simulink model "Bioinspired_backstepping_control"  (R2021b)
settings: Solver=FixedStepAuto  StartTime=0.0  StopTime=10  FixedStep=0.01  RelTol=1e-3
settings Model: Creator=chane  LastModifiedBy=jayeshjayashankar

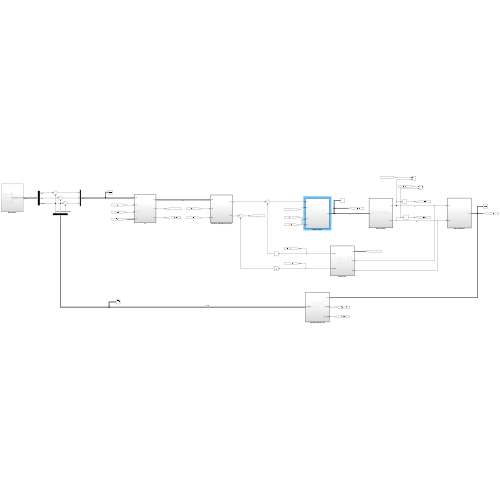
[thumbnail: Simulink's stored preview of the top-level diagram]
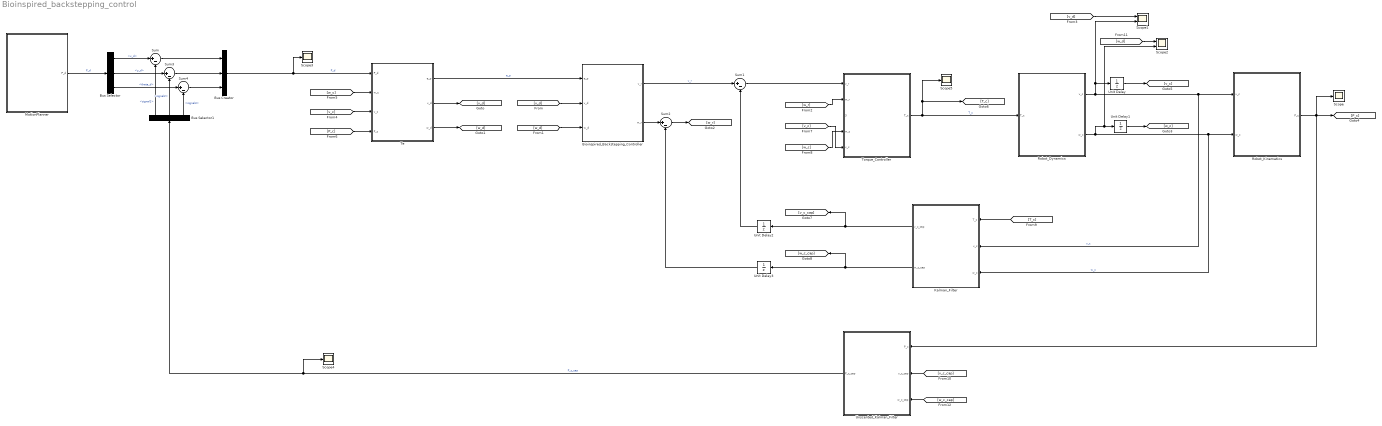
== system Bioinspired_backstepping_control ==
  Bioinspired_Backstepping_Controller : Subsystem  TreatAsAtomicUnit=on
  Bus Creator : BusCreator  Inputs=3
  Bus Selector : BusSelector  OutputSignals=x_d,y_d,theta_d
  Bus Selector1 : BusSelector  OutputSignals=signal1,signal2,signal3
  Kalman_Filter : Subsystem  TreatAsAtomicUnit=on
  MotionPlanner : Subsystem
  Robot_Dynamics : Subsystem  TreatAsAtomicUnit=on
      settings: MinAlgLoopOccurrences=on
  Robot_Kinematics : Subsystem  TreatAsAtomicUnit=on
      settings: MinAlgLoopOccurrences=on
  Scope{,3..5} (4 alike) : Scope
  Scope1 : Scope  NumInputPorts=2
  Scope2 : Scope  NumInputPorts=2
  Sum{,1..4} (5 alike) : Sum  Inputs=|+-
  Te : Subsystem  TreatAsAtomicUnit=on
  Torque_Controller : Subsystem  TreatAsAtomicUnit=on
  Unit Delay{,1..3} (4 alike) : UnitDelay  SampleTime=-1  HasFrameUpgradeWarning=on
  Unscented_Kalman_Filter : Subsystem  TreatAsAtomicUnit=on
      settings: MinAlgLoopOccurrences=on
  wires:
  Te/1(e_p) -> Bioinspired_Backstepping_Controller/1(e_p)  "e_p"
  Te/2(v_d) -> [v_d]
  [v_d] -> Bioinspired_Backstepping_Controller/2(v_d)
  Te/3(w_d) -> [w_d]
  [w_d] -> Bioinspired_Backstepping_Controller/3(w_d)
  [w_r] -> Torque_Controller/2(w_r)
  Torque_Controller/1(T_c) -> Scope5/1, [T_c], Robot_Dynamics/1(T_c)  "T_c"
  Robot_Dynamics/1(v_c) -> Kalman_Filter/2(v_c), Robot_Kinematics/1(v_c), Scope1/2, Unit Delay/1  "v_c"
  [v_c] -> Te/3(v_c)
  [w_c] -> Te/2(w_c)
  [P_c] -> Te/4(P_c)
  [v_c] -> Torque_Controller/5(v_c)
  [w_c] -> Torque_Controller/4(w_c)
  [T_c] -> Kalman_Filter/1(T_c)
  Robot_Dynamics/2(w_c) -> Kalman_Filter/3(w_c), Robot_Kinematics/2(w_c), Scope2/2, Unit Delay1/1  "w_c"
  Bioinspired_Backstepping_Controller/1(v_r) -> Sum1/1  "v_r"
  Sum1/1 -> Torque_Controller/1(v_r)
  Kalman_Filter/1(v_c_cap) -> [v_c_cap], Unit Delay2/1
  Kalman_Filter/2(w_c_cap) -> [w_c_cap], Unit Delay3/1
  [v_c_cap] -> Unscented_Kalman_Filter/2(v_c_cap)
  [w_c_cap] -> Unscented_Kalman_Filter/3(w_c_cap)
  Unscented_Kalman_Filter/1(P_c_cap) -> Scope4/1, Bus Selector1/1  "P_c_cap"
  MotionPlanner/1(P_d) -> Bus Selector/1  "P_d"
  Bus Selector/1 -> Sum/1  "<x_d>"
  Bus Selector1/1 -> Sum/2  "<signal1>"
  Sum/1 -> Bus Creator/1
  Bus Selector/2 -> Sum3/1  "<y_d>"
  Bus Selector1/2 -> Sum3/2  "<signal2>"
  Sum3/1 -> Bus Creator/2
  Bus Selector1/3 -> Sum4/2  "<signal3>"
  Bus Selector/3 -> Sum4/1  "<theta_d>"
  Sum4/1 -> Bus Creator/3
  Bus Creator/1 -> Scope3/1, Te/1(P_d)  "P_d"
  Unit Delay/1 -> [v_c]
  Unit Delay1/1 -> [w_c]
  Robot_Kinematics/1(P_c) -> Unscented_Kalman_Filter/1(P_c), Scope/1, [P_c]
  Unit Delay2/1 -> Sum1/2
  Unit Delay3/1 -> Sum2/2
  [v_d] -> Scope1/1
  [w_d] -> Scope2/1
  Bioinspired_Backstepping_Controller/2(w_r) -> Sum2/1
  Sum2/1 -> [w_r]

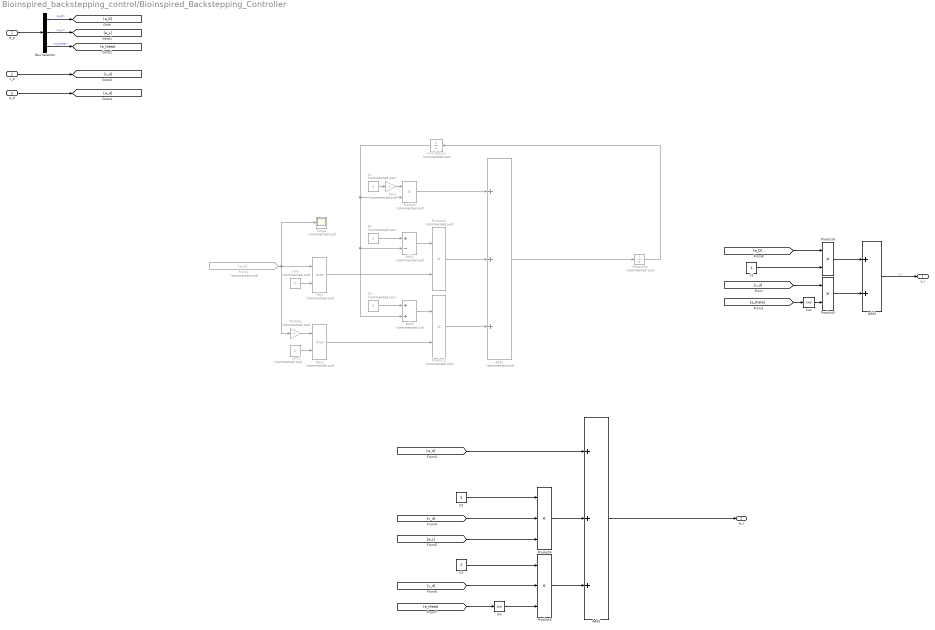
== system Bioinspired_backstepping_control/Bioinspired_Backstepping_Controller ==
  e_p : Inport
  v_d : Inport  Port=2
  w_d : Inport  Port=3
  A1 : Constant  Commented=on  Value=5
  Add1 : Sum  Commented=on  Inputs=+-
  Add2 : Sum  Commented=on
  Add3 : Sum  Commented=on  Inputs=+++
  Add4 : Sum
  Add5 : Sum  Inputs=+++
  B1 : Constant  Commented=on  Value=3
  Bus Selector : BusSelector  OutputSignals=e_D,e_L,e_theta
  C1 : Constant
  C2 : Constant  Value=5
  C3 : Constant  Value=2
  Cos : Trigonometry  Operator=cos
  D1 : Constant  Commented=on  Value=3
  From2 : From  Commented=on  GotoTag=e_D
  Gain : Gain  Commented=on  Gain=-1
  Integrator : Integrator  Commented=on
  Max : MinMax  Commented=on  Function=max  Inputs=2
  Max1 : MinMax  Commented=on  Function=max  Inputs=2
  Multiply : Gain  Commented=on  Gain=-1
  Product : Product  Commented=on
  Product1 : Product  Commented=on
  Product2 : Product  Commented=on
  Product3 : Product
  Product4 : Product  Inputs=3
  Product5 : Product  Inputs=3
  Product6 : Product
  Scope : Scope  Commented=on
  Sin : Trigonometry
  Unit Delay1 : UnitDelay  Commented=on  SampleTime=-1  HasFrameUpgradeWarning=on
  zero : Constant  Commented=on  Value=0
  zero1 : Constant  Commented=on  Value=0
  v_r : Outport
  w_r : Outport  Port=2
  wires:
  e_p/1 -> Bus Selector/1
  Bus Selector/1 -> [e_D]  "<e_D>"
  Bus Selector/2 -> [e_L]  "<e_L>"
  Bus Selector/3 -> [e_theta]  "<e_theta>"
  Add4/1 -> v_r/1  "v_r"
  Integrator/1 -> Unit Delay1/1
  [v_d] -> Product3/1
  Product3/1 -> Add4/2
  D1/1 -> Add2/1
  Max/1 -> Product1/2
  Add3/1 -> Integrator/1
  Add1/1 -> Product1/1
  From2/1 -> Scope/1, Multiply/1, Max/1
  Product1/1 -> Add3/2
  Product/1 -> Add3/1
  Add2/1 -> Product2/1
  [e_theta] -> Cos/1
  Product2/1 -> Add3/3
  zero/1 -> Max/2
  A1/1 -> Gain/1
  Cos/1 -> Product3/2
  Unit Delay1/1 -> Add2/2, Add1/2, Product/2
  B1/1 -> Add1/1
  v_d/1 -> [v_d]
  w_d/1 -> [w_d]
  Add5/1 -> w_r/1
  [w_d] -> Add5/1
  Product4/1 -> Add5/2
  C2/1 -> Product4/1
  [v_d] -> Product4/2
  [e_L] -> Product4/3
  Product5/1 -> Add5/3
  C3/1 -> Product5/1
  [v_d] -> Product5/2
  [e_theta] -> Sin/1
  Sin/1 -> Product5/3
  zero1/1 -> Max1/2
  Max1/1 -> Product2/2
  Multiply/1 -> Max1/1
  Gain/1 -> Product/1
  Product6/1 -> Add4/1
  [e_D] -> Product6/1
  C1/1 -> Product6/2

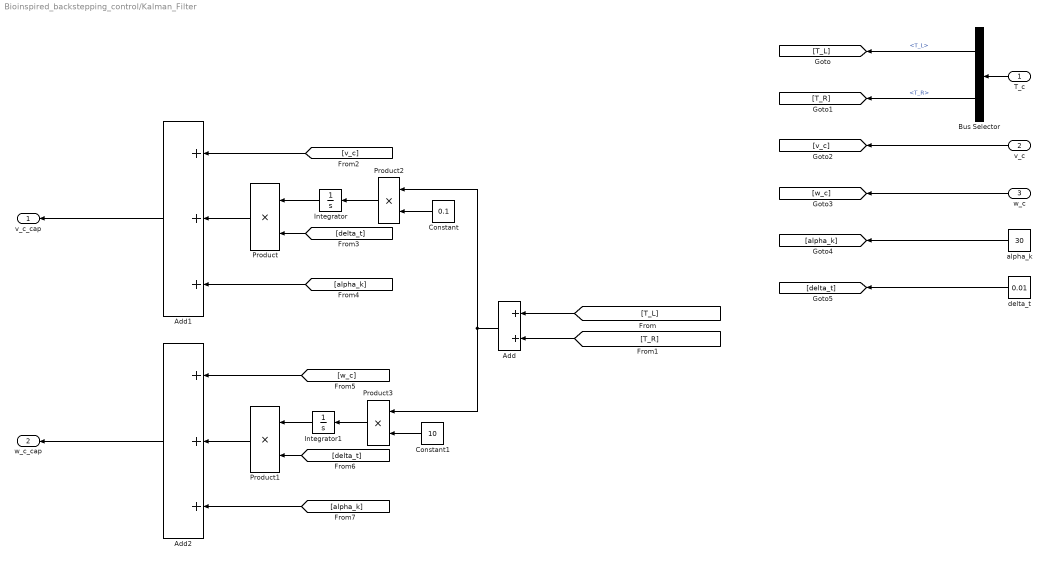
== system Bioinspired_backstepping_control/Kalman_Filter ==
  T_c : Inport
  v_c : Inport  Port=2
  w_c : Inport  Port=3
  Add : Sum
  Add1 : Sum  Inputs=+++
  Add2 : Sum  Inputs=+++
  Bus Selector : BusSelector  OutputSignals=T_L,T_R
  Constant : Constant  Value=0.1
  Constant1 : Constant  Value=10
  Integrator : Integrator
  Integrator1 : Integrator
  Product : Product
  Product1 : Product
  Product2 : Product  Inputs=**
  Product3 : Product  Inputs=**
  alpha_k : Constant  Value=30
  delta_t : Constant  Value=0.01
  v_c_cap : Outport
  w_c_cap : Outport  Port=2
  wires:
  T_c/1 -> Bus Selector/1
  [T_L] -> Add/1
  Constant/1 -> Product2/2
  [T_R] -> Add/2
  [delta_t] -> Product/2
  [v_c] -> Add1/1
  Product/1 -> Add1/2
  [alpha_k] -> Add1/3
  Product1/1 -> Add2/2
  Add/1 -> Product3/1, Product2/1
  [w_c] -> Add2/1
  [delta_t] -> Product1/2
  [alpha_k] -> Add2/3
  Bus Selector/1 -> [T_L]  "<T_L>"
  Bus Selector/2 -> [T_R]  "<T_R>"
  v_c/1 -> [v_c]
  w_c/1 -> [w_c]
  alpha_k/1 -> [alpha_k]
  delta_t/1 -> [delta_t]
  Add1/1 -> v_c_cap/1
  Add2/1 -> w_c_cap/1
  Constant1/1 -> Product3/2
  Product2/1 -> Integrator/1
  Product3/1 -> Integrator1/1
  Integrator/1 -> Product/1
  Integrator1/1 -> Product1/1

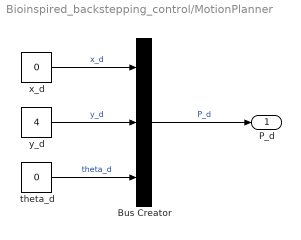
== system Bioinspired_backstepping_control/MotionPlanner ==
  Bus Creator : BusCreator  Inputs=3
  theta_d : Constant  Value=0
  x_d : Constant  Value=0
  y_d : Constant  Value=4
  P_d : Outport
  wires:
  y_d/1 -> Bus Creator/2  "y_d"
  x_d/1 -> Bus Creator/1  "x_d"
  theta_d/1 -> Bus Creator/3  "theta_d"
  Bus Creator/1 -> P_d/1  "P_d"

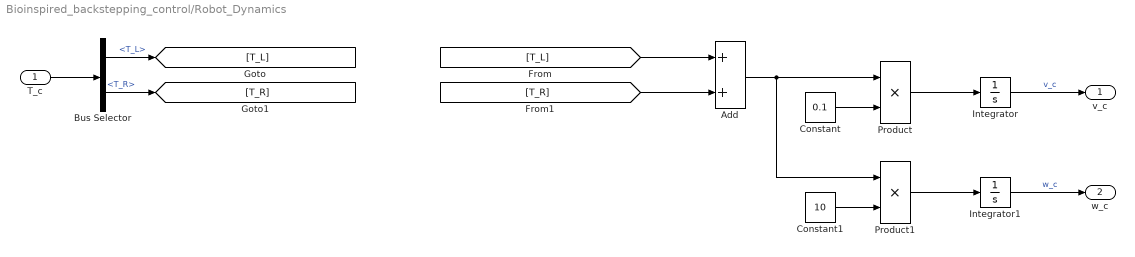
== system Bioinspired_backstepping_control/Robot_Dynamics ==
  T_c : Inport
  Add : Sum
  Bus Selector : BusSelector  OutputSignals=T_L,T_R
  Constant : Constant  Value=0.1
  Constant1 : Constant  Value=10
  Integrator : Integrator
  Integrator1 : Integrator
  Product : Product  Inputs=**
  Product1 : Product  Inputs=**
  v_c : Outport
  w_c : Outport  Port=2
  wires:
  T_c/1 -> Bus Selector/1
  Bus Selector/1 -> [T_L]  "<T_L>"
  Bus Selector/2 -> [T_R]  "<T_R>"
  [T_L] -> Add/1
  [T_R] -> Add/2
  Add/1 -> Product1/1, Product/1
  Constant/1 -> Product/2
  Product/1 -> Integrator/1
  Integrator/1 -> v_c/1  "v_c"
  Integrator1/1 -> w_c/1  "w_c"
  Constant1/1 -> Product1/2
  Product1/1 -> Integrator1/1

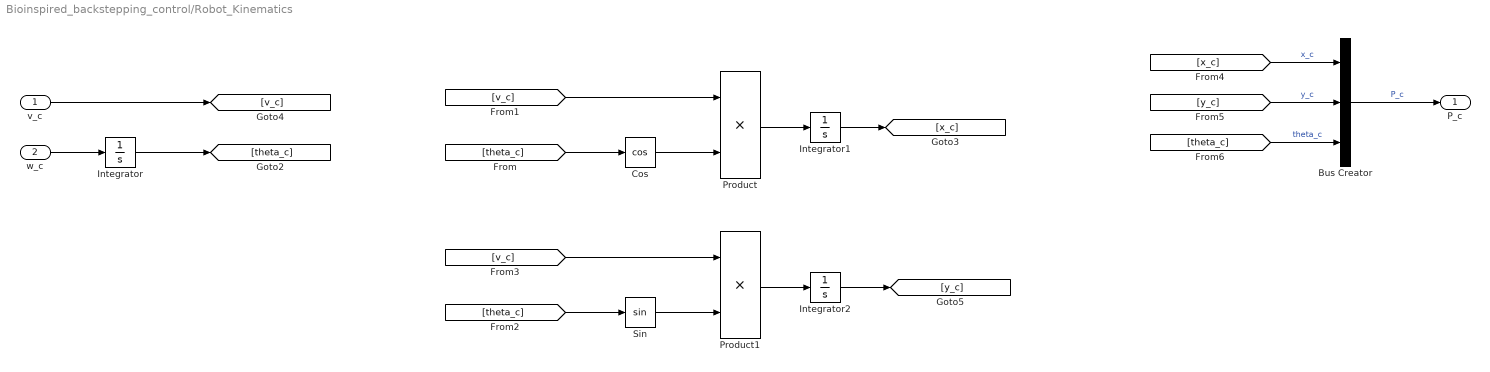
== system Bioinspired_backstepping_control/Robot_Kinematics ==
  v_c : Inport
  w_c : Inport  Port=2
  Bus Creator : BusCreator  Inputs=3
  Cos : Trigonometry  Operator=cos
  Integrator : Integrator
  Integrator1 : Integrator
  Integrator2 : Integrator
  Product : Product
  Product1 : Product
  Sin : Trigonometry
  P_c : Outport
  wires:
  v_c/1 -> [v_c]
  w_c/1 -> Integrator/1
  Integrator/1 -> [theta_c]
  [theta_c] -> Cos/1
  Cos/1 -> Product/2
  [v_c] -> Product/1
  Product/1 -> Integrator1/1
  Integrator1/1 -> [x_c]
  Product1/1 -> Integrator2/1
  Sin/1 -> Product1/2
  [theta_c] -> Sin/1
  [v_c] -> Product1/1
  [x_c] -> Bus Creator/1  "x_c"
  [y_c] -> Bus Creator/2  "y_c"
  [theta_c] -> Bus Creator/3  "theta_c"
  Bus Creator/1 -> P_c/1  "P_c"
  Integrator2/1 -> [y_c]

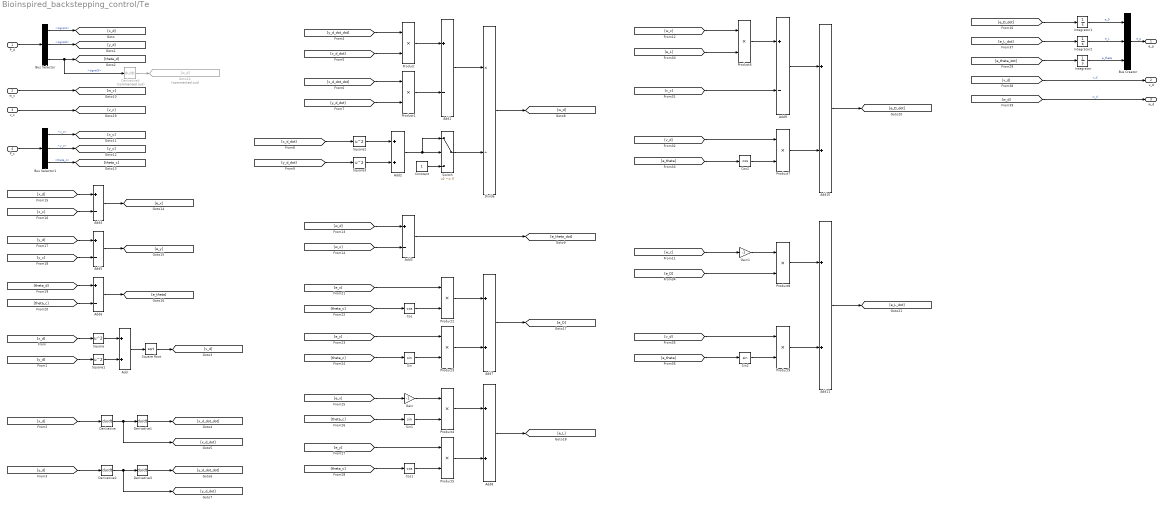
== system Bioinspired_backstepping_control/Te ==
  P_d : Inport
  w_c : Inport  Port=2
  v_c : Inport  Port=3
  P_c : Inport  Port=4
  Add{,7..8,10..11} (5 alike) : Sum
  Add{1,3..6,9} (6 alike) : Sum  Inputs=+-
  Add2 : Sum  OutMin=0.1
  Bus Creator : BusCreator  Inputs=3
  Bus Selector : BusSelector  OutputSignals=signal1,signal2,signal3
  Bus Selector1 : BusSelector  OutputSignals=x_c,y_c,theta_c
  Constant : Constant
  Cos : Trigonometry  Operator=cos
  Cos1 : Trigonometry  Operator=cos
  Cos2 : Trigonometry  Operator=cos
  Derivative{,1..3} (4 alike) : Derivative
  Derivative4 : Derivative  Commented=on
  Divide : Product  Inputs=*/
  Gain : Gain  Gain=-1
  Gain1 : Gain  Gain=-1
  Goto22 : Goto  Commented=on  GotoTag=w_d
  Integrator : Integrator
  Integrator1 : Integrator
  Integrator2 : Integrator
  Product{,1..9} (10 alike) : Product
  Sin : Trigonometry
  Sin1 : Trigonometry
  Sin2 : Trigonometry
  Square{,1..3} (4 alike) : Math  Operator=square  SaturateOnIntegerOverflow=on
  Square Root : Sqrt  SaturateOnIntegerOverflow=on
  Switch : Switch  Criteria=u2 ~= 0
  e_p : Outport
  v_d : Outport  Port=2
  w_d : Outport  Port=3
  wires:
  Bus Creator/1 -> e_p/1  "e_p"
  P_d/1 -> Bus Selector/1
  Bus Selector/1 -> [x_d]  "<signal1>"
  Bus Selector/2 -> [y_d]  "<signal2>"
  Bus Selector/3 -> Derivative4/1, [theta_d]  "<signal3>"
  [x_d] -> Square/1
  [y_d] -> Square1/1
  Square1/1 -> Add/2
  Square/1 -> Add/1
  Add/1 -> Square Root/1
  Square Root/1 -> [v_d]
  [x_d] -> Derivative/1
  Derivative/1 -> [x_d_dot], Derivative1/1
  Derivative1/1 -> [x_d_dot_dot]
  Derivative3/1 -> [y_d_dot_dot]
  Derivative2/1 -> Derivative3/1, [y_d_dot]
  [y_d] -> Derivative2/1
  [y_d_dot_dot] -> Product/1
  [x_d_dot] -> Product/2
  [x_d_dot_dot] -> Product1/1
  [y_d_dot] -> Product1/2
  Product/1 -> Add1/1
  Product1/1 -> Add1/2
  [x_d_dot] -> Square2/1
  [y_d_dot] -> Square3/1
  Square2/1 -> Add2/1
  Square3/1 -> Add2/2
  Add1/1 -> Divide/1
  Divide/1 -> [w_d]
  Integrator1/1 -> Bus Creator/1  "e_D"
  Integrator/1 -> Bus Creator/3  "e_theta"
  [w_d] -> Add3/1
  Add3/1 -> [e_theta_dot]
  [w_c] -> Add3/2
  [x_d] -> Add4/1
  [x_c] -> Add4/2
  [y_d] -> Add5/1
  [y_c] -> Add5/2
  [theta_d] -> Add6/1
  [theta_c] -> Add6/2
  Add4/1 -> [e_x]
  Add5/1 -> [e_y]
  Add6/1 -> [e_theta]
  [theta_c] -> Cos/1
  [e_x] -> Product2/1
  Cos/1 -> Product2/2
  [e_y] -> Product3/1
  Sin/1 -> Product3/2
  [theta_c] -> Sin/1
  Product2/1 -> Add7/1
  Product3/1 -> Add7/2
  Add7/1 -> [e_D]
  Product5/1 -> Add8/2
  Product4/1 -> Add8/1
  [theta_c] -> Cos1/1
  Cos1/1 -> Product5/2
  [e_y] -> Product5/1
  Sin1/1 -> Product4/2
  [e_x] -> Gain/1
  [theta_c] -> Sin1/1
  Gain/1 -> Product4/1
  Add8/1 -> [e_L]
  [e_theta_dot] -> Integrator/1
  [w_c] -> Product6/1
  [e_L] -> Product6/2
  Product6/1 -> Add9/1
  [v_c] -> Add9/2
  Add9/1 -> Add10/1
  Cos2/1 -> Product7/2
  [v_d] -> Product7/1
  Product7/1 -> Add10/2
  [e_theta] -> Cos2/1
  Add10/1 -> [e_D_dot]
  [e_D_dot] -> Integrator1/1
  Integrator2/1 -> Bus Creator/2  "e_L"
  [w_c] -> Gain1/1
  [e_D] -> Product8/2
  Gain1/1 -> Product8/1
  Product8/1 -> Add11/1
  Product9/1 -> Add11/2
  [v_d] -> Product9/1
  Sin2/1 -> Product9/2
  [e_theta] -> Sin2/1
  Add11/1 -> [e_L_dot]
  [e_L_dot] -> Integrator2/1
  [v_d] -> v_d/1  "v_d"
  [w_d] -> w_d/1  "w_d"
  w_c/1 -> [w_c]
  v_c/1 -> [v_c]
  Bus Selector1/1 -> [x_c]  "<x_c>"
  Bus Selector1/2 -> [y_c]  "<y_c>"
  Bus Selector1/3 -> [theta_c]  "<theta_c>"
  P_c/1 -> Bus Selector1/1
  Add2/1 -> Switch/1, Switch/2
  Switch/1 -> Divide/2
  Constant/1 -> Switch/3
  Derivative4/1 -> Goto22/1

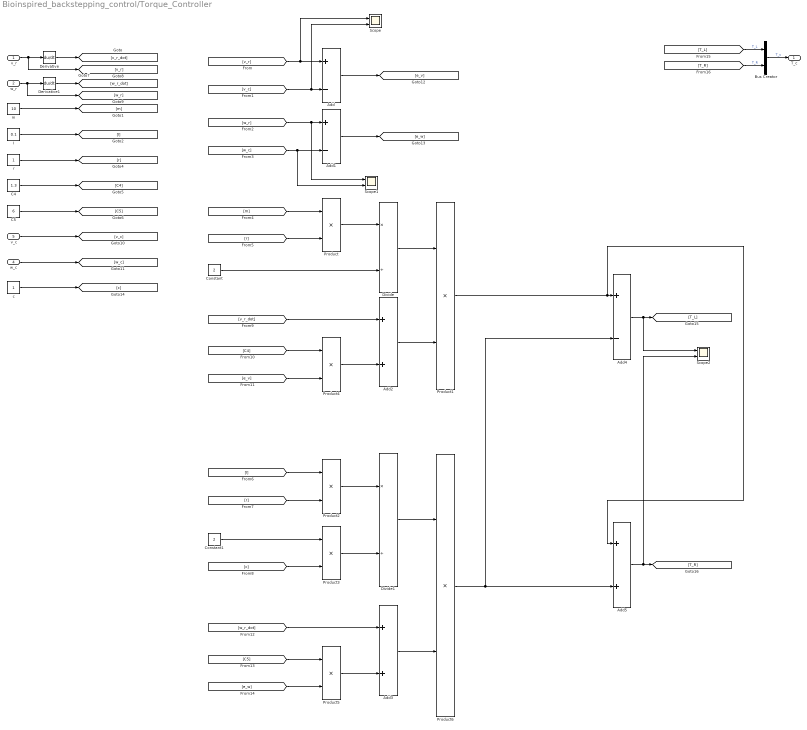
== system Bioinspired_backstepping_control/Torque_Controller ==
  v_r : Inport
  w_r : Inport  Port=2
  w_c : Inport  Port=4
  v_c : Inport  Port=5
  Add : Sum  Inputs=+-
  Add1 : Sum  Inputs=+-
  Add2 : Sum
  Add3 : Sum
  Add4 : Sum  Inputs=+-
  Add5 : Sum
  Bus Creator : BusCreator  Inputs=2
  C4 : Constant  Value=1.3
  C5 : Constant  Value=6
  Constant : Constant  Value=2
  Constant1 : Constant  Value=2
  Derivative : Derivative
  Derivative1 : Derivative
  Divide : Product  Inputs=*/
  Divide1 : Product  Inputs=*/
  I : Constant  Value=0.1
  Product{,1..6} (7 alike) : Product
  Scope : Scope  NumInputPorts=2
  Scope1 : Scope  NumInputPorts=2
  Scope2 : Scope  NumInputPorts=2
  c : Constant
  m : Constant  Value=10
  r : Constant
  T_c : Outport
  wires:
  v_r/1 -> [v_r], Derivative/1
  Derivative/1 -> [v_r_dot]
  m/1 -> [m]
  I/1 -> [I]
  r/1 -> [r]
  C4/1 -> [C4]
  C5/1 -> [C5]
  Derivative1/1 -> [w_r_dot]
  w_r/1 -> [w_r], Derivative1/1
  [v_r] -> Scope/1, Add/1
  [v_c] -> Scope/2, Add/2
  Add/1 -> [e_v]
  Add1/1 -> [e_w]
  [w_c] -> Scope1/2, Add1/2
  [w_r] -> Scope1/1, Add1/1
  [m] -> Product/1
  [r] -> Product/2
  Product/1 -> Divide/1
  Constant/1 -> Divide/2
  Divide/1 -> Product1/1
  Product2/1 -> Divide1/1
  Product3/1 -> Divide1/2
  [I] -> Product2/1
  [r] -> Product2/2
  c/1 -> [c]
  Constant1/1 -> Product3/1
  [c] -> Product3/2
  Add2/1 -> Product1/2
  [v_r_dot] -> Add2/1
  Product4/1 -> Add2/2
  [C4] -> Product4/1
  [e_v] -> Product4/2
  Product5/1 -> Add3/2
  [e_w] -> Product5/2
  [C5] -> Product5/1
  [w_r_dot] -> Add3/1
  Divide1/1 -> Product6/1
  Add3/1 -> Product6/2
  Product6/1 -> Add4/2, Add5/2
  Product1/1 -> Add5/1, Add4/1
  Add4/1 -> Scope2/1, [T_L]
  Add5/1 -> Scope2/2, [T_R]
  [T_L] -> Bus Creator/1  "T_L"
  [T_R] -> Bus Creator/2  "T_R"
  Bus Creator/1 -> T_c/1  "T_c"
  v_c/1 -> [v_c]
  w_c/1 -> [w_c]

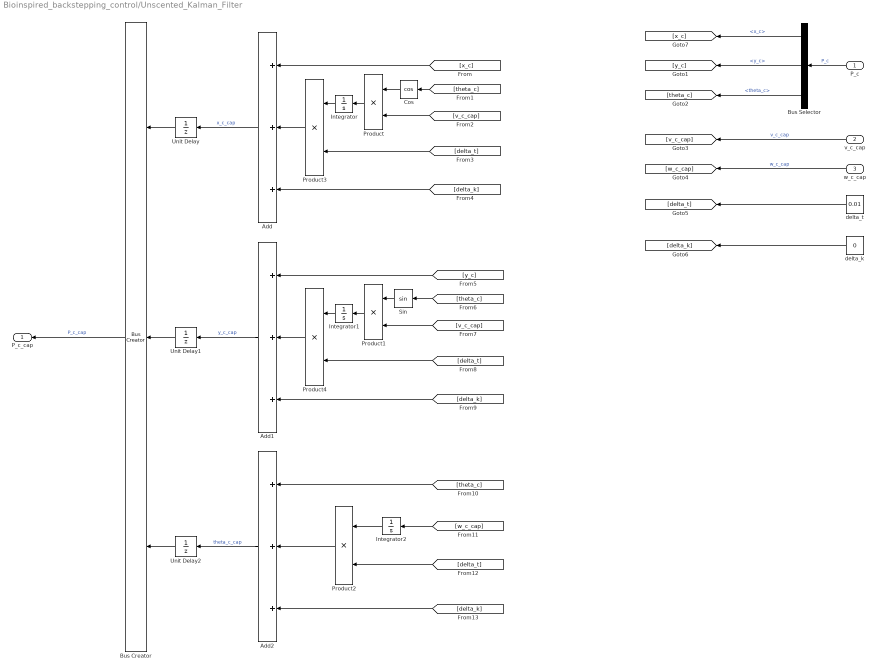
== system Bioinspired_backstepping_control/Unscented_Kalman_Filter ==
  P_c : Inport
  v_c_cap : Inport  Port=2
  w_c_cap : Inport  Port=3
  Add : Sum  Inputs=+++
  Add1 : Sum  Inputs=+++
  Add2 : Sum  Inputs=+++
  Bus Creator : BusCreator  Inputs=3
  Bus Selector : BusSelector  OutputSignals=x_c,y_c,theta_c
  Cos : Trigonometry  Operator=cos
  Integrator : Integrator
  Integrator1 : Integrator
  Integrator2 : Integrator
  Product{,1..4} (5 alike) : Product
  Sin : Trigonometry
  Unit Delay : UnitDelay  SampleTime=-1  HasFrameUpgradeWarning=on
  Unit Delay1 : UnitDelay  SampleTime=-1  HasFrameUpgradeWarning=on
  Unit Delay2 : UnitDelay  SampleTime=-1  HasFrameUpgradeWarning=on
  delta_k : Constant  Value=0
  delta_t : Constant  Value=0.01
  P_c_cap : Outport
  wires:
  P_c/1 -> Bus Selector/1  "P_c"
  Bus Selector/1 -> [x_c]  "<x_c>"
  Bus Selector/2 -> [y_c]  "<y_c>"
  Bus Selector/3 -> [theta_c]  "<theta_c>"
  v_c_cap/1 -> [v_c_cap]  "v_c_cap"
  w_c_cap/1 -> [w_c_cap]  "w_c_cap"
  delta_t/1 -> [delta_t]
  delta_k/1 -> [delta_k]
  [x_c] -> Add/1
  [theta_c] -> Cos/1
  Cos/1 -> Product/1
  [v_c_cap] -> Product/2
  [delta_t] -> Product3/2
  [delta_k] -> Add/3
  [y_c] -> Add1/1
  [theta_c] -> Sin/1
  [delta_k] -> Add1/3
  [theta_c] -> Add2/1
  Product2/1 -> Add2/2
  [delta_t] -> Product2/2
  [delta_k] -> Add2/3
  Add1/1 -> Unit Delay1/1  "y_c_cap"
  Add/1 -> Unit Delay/1  "x_c_cap"
  Bus Creator/1 -> P_c_cap/1  "P_c_cap"
  Add2/1 -> Unit Delay2/1  "theta_c_cap"
  Unit Delay/1 -> Bus Creator/1
  Unit Delay1/1 -> Bus Creator/2
  Unit Delay2/1 -> Bus Creator/3
  Product4/1 -> Add1/2
  Product3/1 -> Add/2
  Product/1 -> Integrator/1
  Product1/1 -> Integrator1/1
  Sin/1 -> Product1/1
  [v_c_cap] -> Product1/2
  [delta_t] -> Product4/2
  [w_c_cap] -> Integrator2/1
  Integrator/1 -> Product3/1
  Integrator1/1 -> Product4/1
  Integrator2/1 -> Product2/1
